simulink model "f16_hifi_euler_vTrim"  (R2020b)
settings: Solver=ode4  StartTime=0.0  StopTime=simTime  FixedStep=stepTime  RelTol=1e-3
undefined symbols (not defined in the file): data, ft, outputs, s
libraries: libAeroLookUpTables x9, aerolibconvert2 x7, lib6DOFUtilityEquations x6, libTFActuatorCalc x5, aerolibtransform2 x1, libEngineAngMomSpecs x1, libAircraftMoISpecs x1, libAircraftWeightandMassSpec x1, libAircraftWingFusalageSpecs x1, libCmdPowConversion x1, libEngineThrustCalc x1, libAtmosphereModel x1
(part 2 of 3)

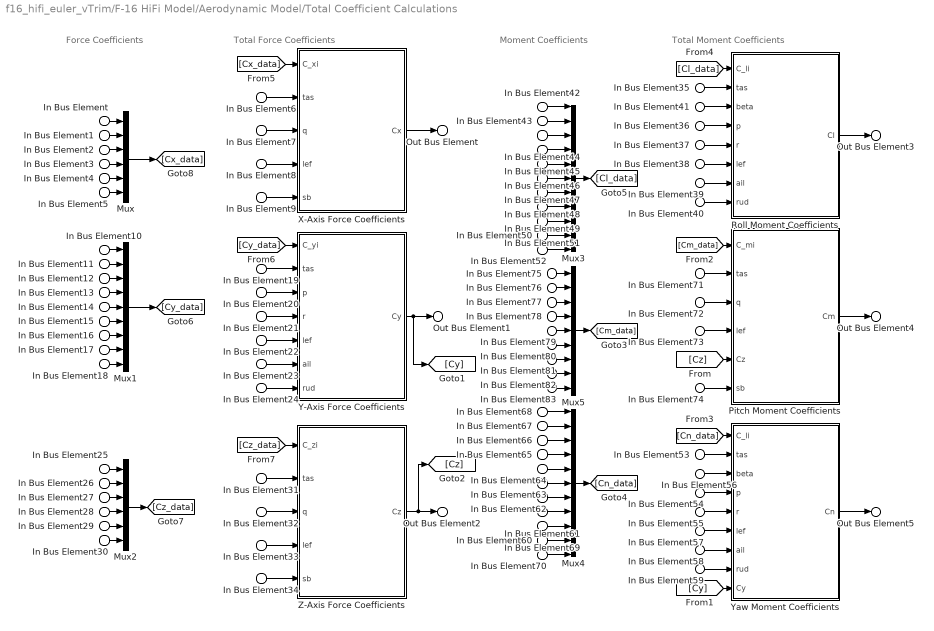
== system f16_hifi_euler_vTrim/F-16 HiFi Model/Aerodynamic Model/Total Coefficient Calculations ==
  note: Total Moment Coefficients
  note: Total Force Coefficients
  note: Force Coefficients
  note: Moment Coefficients
  In Bus Element : Inport  PortName=coeffs  Element=Cx
  In Bus Element1 : Inport  PortName=coeffs  Element=Cxq
  In Bus Element2 : Inport  PortName=coeffs  Element=Cxlef
  In Bus Element3 : Inport  PortName=coeffs  Element=Cxqlef
  In Bus Element4 : Inport  PortName=coeffs  Element=Cxsb
  In Bus Element5 : Inport  PortName=coeffs  Element=Cx0
  In Bus Element10 : Inport  PortName=coeffs  Element=Cy
  In Bus Element11 : Inport  PortName=coeffs  Element=Cyp
  In Bus Element12 : Inport  PortName=coeffs  Element=Cyr
  In Bus Element13 : Inport  PortName=coeffs  Element=Cyail
  In Bus Element14 : Inport  PortName=coeffs  Element=Cyrud
  In Bus Element15 : Inport  PortName=coeffs  Element=Cylef
  In Bus Element16 : Inport  PortName=coeffs  Element=Cyplef
  In Bus Element17 : Inport  PortName=coeffs  Element=Cyrlef
  In Bus Element18 : Inport  PortName=coeffs  Element=Cyaillef
  In Bus Element25 : Inport  PortName=coeffs  Element=Cz
  In Bus Element26 : Inport  PortName=coeffs  Element=Czq
  In Bus Element27 : Inport  PortName=coeffs  Element=Czlef
  In Bus Element28 : Inport  PortName=coeffs  Element=Czqlef
  In Bus Element29 : Inport  PortName=coeffs  Element=Czsb
  In Bus Element30 : Inport  PortName=coeffs  Element=Cz0
  In Bus Element50 : Inport  PortName=coeffs  Element=Claillef
  In Bus Element49 : Inport  PortName=coeffs  Element=Clrlef
  In Bus Element48 : Inport  PortName=coeffs  Element=Clplef
  In Bus Element47 : Inport  PortName=coeffs  Element=Cllef
  In Bus Element46 : Inport  PortName=coeffs  Element=Clrud
  In Bus Element45 : Inport  PortName=coeffs  Element=Clail
  In Bus Element44 : Inport  PortName=coeffs  Element=Clr
  In Bus Element43 : Inport  PortName=coeffs  Element=Clp
  In Bus Element42 : Inport  PortName=coeffs  Element=Cl
  In Bus Element51 : Inport  PortName=coeffs  Element=Clbeta
  In Bus Element52 : Inport  PortName=coeffs  Element=Cl0
  In Bus Element70 : Inport  PortName=coeffs  Element=Cn0
  In Bus Element60 : Inport  PortName=coeffs  Element=Cnaillef
  In Bus Element69 : Inport  PortName=coeffs  Element=Cnbeta
  In Bus Element61 : Inport  PortName=coeffs  Element=Cnrlef
  In Bus Element62 : Inport  PortName=coeffs  Element=Cnplef
  In Bus Element63 : Inport  PortName=coeffs  Element=Cnlef
  In Bus Element64 : Inport  PortName=coeffs  Element=Cnrud
  In Bus Element65 : Inport  PortName=coeffs  Element=Cnail
  In Bus Element66 : Inport  PortName=coeffs  Element=Cnr
  In Bus Element67 : Inport  PortName=coeffs  Element=Cnp
  In Bus Element75 : Inport  PortName=coeffs  Element=Cm
  In Bus Element76 : Inport  PortName=coeffs  Element=Cmq
  In Bus Element77 : Inport  PortName=coeffs  Element=Cmlef
  In Bus Element78 : Inport  PortName=coeffs  Element=Cmqlef
  In Bus Element79 : Inport  PortName=coeffs  Element=Cmeta
  In Bus Element80 : Inport  PortName=coeffs  Element=Cmdiff
  In Bus Element81 : Inport  PortName=coeffs  Element=Cmds
  In Bus Element82 : Inport  PortName=coeffs  Element=Cmsb
  In Bus Element83 : Inport  PortName=coeffs  Element=Cm0
  In Bus Element68 : Inport  PortName=coeffs  Element=Cn
  In Bus Element{6,19,31,35,53,71} (6 alike) : Inport  Port=2  PortName=states  Element=tas
  In Bus Element7 : Inport  Port=2  PortName=states  Element=q
  In Bus Element32 : Inport  Port=2  PortName=states  Element=q
  In Bus Element72 : Inport  Port=2  PortName=states  Element=q
  In Bus Element20 : Inport  Port=2  PortName=states  Element=p
  In Bus Element36 : Inport  Port=2  PortName=states  Element=p
  In Bus Element54 : Inport  Port=2  PortName=states  Element=p
  In Bus Element21 : Inport  Port=2  PortName=states  Element=r
  In Bus Element37 : Inport  Port=2  PortName=states  Element=r
  In Bus Element55 : Inport  Port=2  PortName=states  Element=r
  In Bus Element41 : Inport  Port=2  PortName=states  Element=beta
  In Bus Element56 : Inport  Port=2  PortName=states  Element=beta
  In Bus Element{8,22,33,38,57,73} (6 alike) : Inport  Port=3  PortName=actSignals  Element=lef
  In Bus Element9 : Inport  Port=3  PortName=actSignals  Element=sb
  In Bus Element34 : Inport  Port=3  PortName=actSignals  Element=sb
  In Bus Element74 : Inport  Port=3  PortName=actSignals  Element=sb
  In Bus Element23 : Inport  Port=3  PortName=actSignals  Element=ail
  In Bus Element39 : Inport  Port=3  PortName=actSignals  Element=ail
  In Bus Element58 : Inport  Port=3  PortName=actSignals  Element=ail
  In Bus Element24 : Inport  Port=3  PortName=actSignals  Element=rud
  In Bus Element40 : Inport  Port=3  PortName=actSignals  Element=rud
  In Bus Element59 : Inport  Port=3  PortName=actSignals  Element=rud
  Mux : Mux  Inputs=6
  Mux1 : Mux  Inputs=09
  Mux2 : Mux  Inputs=6
  Mux3 : Mux  Inputs=11
  Mux4 : Mux  Inputs=11
  Mux5 : Mux  Inputs=09
  Pitch Moment Coefficients : Subsystem  mask(Aerodynamic Model -> Total Coefficient Calculations -> Total Pitch Moment Body Aerodynamic Coefficient){cbar=data.acSpec.wing.cbar, xcg=data.acSpec.fusalage.x_cg, xcg_ref=data.acSpec.fusalage.x_cg_ref}
      mask prompts: cbar "Mean Aerodynamic Chord"; xcg "X-axis center of gravity"; xcg_ref "Nominal X-axis center of gravity"
      mask help:
      | Total Pitch Moment Body Aerodynamic Coefficient Calculatior.
      | Aircraft state information and control inputs are used for calculations.
      mask Help:
      | This block is used for obtain total pitch moment coefficient with using state and control inputs.
      | -------------------------------------------------------------------------------------------------------------------------------------------------
      | Inputs of the function:
      | 	Coefficients C_{m}s: Pitch Moment whole aerodynamic coefficients at specific conditions.
      | 	tas: True air speed in [ft/s].
      | 	q: Body axis angular rate (pitch) in [rad/s].
      | 	lef: Leading edge flap deflection in [deg].
      | 	C_{z}: Z-Axis total aeodynamic coefficient.
      | Output of the function:
      | 	C_{m}: Pitch Moment total aerodynamic coefficient.
      | -------------------------------------------------------------------------------------------------------------------------------------------------
      | 	- All equations can be found in Steven's text book. Reference can be found in "literature" subfolder.
      | 	- for question: "cagataysahin44@gmail.com"
      mask Display:
      | port_label('input',1,'C_{m_{i}}','texmode','on');
      | port_label('input',2,'V_{tas}','texmode','on');
      | port_label('input',3,'q','texmode','on');
      | port_label('input',4,'\delta_{lef}','texmode','on');
      | port_label('input',5,'C_{z}','texmode','on');
      | port_label('input',6,'\delta_{sb}','texmode','on');
      | 
      | port_label('output',1,'C_{m}','texmode','on');
  Roll Moment Coefficients : Subsystem  mask(Aerodynamic Model -> Total Coefficient Calculations -> Total Roll Moment Body Aerodynamic Coefficient){b=data.acSpec.wing.b}
      mask prompts: b "Wing Span"
      mask help:
      | Total Roll Moment Aerodynamic Coefficient Calculatior.
      | Aircraft state information and control inputs are used for calculations.
      mask Help:
      | This block is used for obtain total roll moment aerodynamic force coefficient. The equations are taken from Steven's textbook.,
      | -------------------------------------------------------------------------------------------------------------------------------------------------
      | Inputs of the function:
      | 	Coefficients C_{l}s: Roll moment whole aerodynamic coefficients at specific conditions.
      | 	tas: True air speed in [ft/s].
      |  	beta: Sideslip angle in [rad].
      | 	p: Body axis angular rate (roll) in [rad/s].
      | 	r: Body axis angular rate (yaw) in [rad/s].
      | 	lef: Leading edge flap deflection in [deg].
      | 	ail: Aileron deflection in [deg].
      | 	rud: Rudder deflection in [deg].
      | Output of the function:
      | 	C_{l}: Roll moment aerodynamic coefficient.
      | -------------------------------------------------------------------------------------------------------------------------------------------------
      | 	- All equations can be found in Steven's text book. Reference can be found in "literature" subfolder.
      | 	- for question: "cagataysahin44@gmail.com"
      mask Display:
      | port_label('input',1,'C_{l_{i}}','texmode','on');
      | port_label('input',2,'V_{tas}','texmode','on');
      | port_label('input',3,'\beta','texmode','on');
      | port_label('input',4,'p','texmode','on');
      | port_label('input',5,'r','texmode','on');
      | port_label('input',6,'\delta_{lef}','texmode','on');
      | port_label('input',7,'\delta_{ail}','texmode','on');
      | port_label('input',8,'\delta_{rud}','texmode','on');
      | 
      | port_label('output',1,'C_{l}','texmode','on');
  X-Axis Force Coefficients : Subsystem  mask(Aerodynamic Model -> Total Coefficient Calculations -> Total X-Axis Body Aerodynamic Coefficient){cbar=data.acSpec.wing.cbar}
      mask prompts: cbar "Mean Aerodynamic Chord"
      mask help:
      | Total X-Axis Body Aerodynamic Coefficient Calculatior.
      | Aircraft state information and control inputs are used for calculations.
      mask Help:
      | This block is used for obtain total x-axis aerodynamic force coefficient with using state and control inputs.
      | -------------------------------------------------------------------------------------------------------------------------------------------------
      | Inputs of the function:
      | 	Coefficients C_{x}s: X-Axis whole aerodynamic coefficients at specific conditions.
      | 	tas: True air speed in [ft/s].
      | 	q: Body axis angular rate (pitch) in [rad/s].
      | 	lef: Leading edge flap deflection in [deg].
      | Output of the function:
      | 	C_{x}: X-Axis total aerodynamic coefficient.
      | -------------------------------------------------------------------------------------------------------------------------------------------------
      | 	- All equations can be found in Steven's text book. Reference can be found in "literature" subfolder.
      | 	- for question: "cagataysahin44@gmail.com"
      mask Display:
      | port_label('input',1,'C_{x_{i}}','texmode','on');
      | port_label('input',2,'V_{tas}','texmode','on');
      | port_label('input',3,'q','texmode','on');
      | port_label('input',4,'\delta_{lef}','texmode','on');
      | port_label('input',5,'\delta_{sb}','texmode','on');
      | 
      | port_label('output',1,'C_{x}','texmode','on');
  Y-Axis Force Coefficients : Subsystem  mask(Aerodynamic Model -> Total Coefficient Calculations -> Total Y-Axis Body Aerodynamic Coefficient){b=data.acSpec.wing.b}
      mask prompts: b "Wing Span"
      mask help:
      | Total Y-Axis Body Aerodynamic Coefficient Calculatior.
      | Aircraft state information and control inputs are used for calculations.
      mask Help:
      | This block is used for obtain total x-axis aerodynamic force coefficient with using state and control inputs.
      | -------------------------------------------------------------------------------------------------------------------------------------------------
      | Inputs of the function:
      | 	Coefficients C_{y}s: Y-Axis whole aerodynamic coefficients at specific conditions.
      | 	tas: True air speed in [ft/s].
      | 	p: Body axis angular rate (y-axis) in [rad/s].
      | 	r: Body axis angular rate (y-axis) in [rad/s].
      | 	lef: Leading edge flap deflection in [deg].
      | 	ail: Aileron deflection in [deg].
      | 	rud: Rudder deflection in [deg].
      | Output of the function:
      | 	C_{y}: Y-axis total aerodynamic coefficient.
      | -------------------------------------------------------------------------------------------------------------------------------------------------
      | 	- All equations can be found in Steven's text book. Reference can be found in "literature" subfolder.
      | 	- for question: "cagataysahin44@gmail.com"
      mask Display:
      | port_label('input',1,'C_{y_{i}}','texmode','on');
      | port_label('input',2,'V_{tas}','texmode','on');
      | port_label('input',3,'p','texmode','on');
      | port_label('input',4,'r','texmode','on');
      | port_label('input',5,'\delta_{lef}','texmode','on');
      | port_label('input',6,'\delta_{ail}','texmode','on');
      | port_label('input',7,'\delta_{rud}','texmode','on');
      | 
      | port_label('output',1,'C_{y}','texmode','on');
  Yaw Moment Coefficients : Subsystem  mask(Aerodynamic Model -> Total Coefficient Calculations -> Total Yaw Moment Body Aerodynamic Coefficient){b=data.acSpec.wing.b, xcg=data.acSpec.fusalage.x_cg, xcg_ref=data.acSpec.fusalage.x_cg_ref, cbar=data.acSpec.wing.cbar}
      mask prompts: b "Wing Span"; xcg "Center of Gravity"; xcg_ref "Nominal Center of Gravity"; cbar "Mean Aerodynamic Chord"
      mask help:
      | Total Yaw Moment Aerodynamic Coefficient Calculatior.
      | Aircraft state information and control inputs are used for calculations.
      mask Help:
      | This block is used for obtain total yaw moment aerodynamic force coefficient. The equations are taken from Steven's textbook.,
      | -------------------------------------------------------------------------------------------------------------------------------------------------
      | Inputs of the function:
      | 	Coefficients C_{n}s: Yaw moment whole aerodynamic coefficients at specific conditions.
      | 	tas: True air speed in [ft/s].
      |  	beta: Sideslip angle in [rad].
      | 	p: Body axis angular rate (roll) in [rad/s].
      | 	r: Body axis angular rate (yaw) in [rad/s].
      | 	lef: Leading edge flap deflection in [deg].
      | 	ail: Aileron deflection in [deg].
      | 	rud: Rudder deflection in [deg].
      | 	C_{y}: Total Y-Axis aerodynamic coefficient.
      | Output of the function:
      | 	C_{n}: Yaw moment aerodynamic coefficient.
      | -------------------------------------------------------------------------------------------------------------------------------------------------
      | 	- All equations can be found in Steven's text book. Reference can be found in "literature" subfolder.
      | 	- for question: "cagataysahin44@gmail.com"
      mask Display:
      | port_label('input',1,'C_{n_{i}}','texmode','on');
      | port_label('input',2,'V_{tas}','texmode','on');
      | port_label('input',3,'\beta','texmode','on');
      | port_label('input',4,'p','texmode','on');
      | port_label('input',5,'r','texmode','on');
      | port_label('input',6,'\delta_{lef}','texmode','on');
      | port_label('input',7,'\delta_{ail}','texmode','on');
      | port_label('input',8,'\delta_{rud}','texmode','on');
      | port_label('input',9,'C_{y}','texmode','on');
      | 
      | port_label('output',1,'C_{n}','texmode','on');
  Z-Axis Force Coefficients : Subsystem  mask(Aerodynamic Model -> Total Coefficient Calculations -> Total Z-Axis Body Aerodynamic Coefficient){cbar=data.acSpec.wing.cbar}
      mask prompts: cbar "Mean Aerodynamic Chord"
      mask help:
      | Total Z-Axis Body Aerodynamic Coefficient Calculatior.
      | Aircraft state information and control inputs are used for calculations.
      mask Help:
      | This block is used for obtain total z-axis aerodynamic force coefficient with using state and control inputs.
      | -------------------------------------------------------------------------------------------------------------------------------------------------
      | Inputs of the function:
      | 	Coefficients C_{z}s: Z-Axis whole aerodynamic coefficients at specific conditions.
      | 	tas: True air speed in [ft/s].
      | 	q: Body axis angular rate (pitch) in [rad/s].
      | 	lef: Leading edge flap deflection in [deg].
      | Output of the function:
      | 	C_{z}: X-Axis total aerodynamic coefficient.
      | -------------------------------------------------------------------------------------------------------------------------------------------------
      | 	- All equations can be found in Steven's text book. Reference can be found in "literature" subfolder.
      | 	- for question: "cagataysahin44@gmail.com"
      mask Display:
      | port_label('input',1,'C_{z_{i}}','texmode','on');
      | port_label('input',2,'V_{tas}','texmode','on');
      | port_label('input',3,'q','texmode','on');
      | port_label('input',4,'\delta_{lef}','texmode','on');
      | port_label('input',5,'\delta_{sb}','texmode','on');
      | 
      | port_label('output',1,'C_{z}','texmode','on');
  Out Bus Element : Outport  PortName=totalCoeffs  Element=Cx
  Out Bus Element1 : Outport  PortName=totalCoeffs  Element=Cy
  Out Bus Element2 : Outport  PortName=totalCoeffs  Element=Cz
  Out Bus Element3 : Outport  PortName=totalCoeffs  Element=Cl
  Out Bus Element4 : Outport  PortName=totalCoeffs  Element=Cm
  Out Bus Element5 : Outport  PortName=totalCoeffs  Element=Cn
  wires:
  In Bus Element17/1 -> Mux1/8
  In Bus Element78/1 -> Mux5/4
  X-Axis Force Coefficients/1(Cx) -> Out Bus Element/1
  In Bus Element74/1 -> Pitch Moment Coefficients/6(sb)
  In Bus Element23/1 -> Y-Axis Force Coefficients/6(ail)
  In Bus Element7/1 -> X-Axis Force Coefficients/3(q)
  In Bus Element83/1 -> Mux5/9
  In Bus Element68/1 -> Mux4/1
  In Bus Element80/1 -> Mux5/6
  In Bus Element35/1 -> Roll Moment Coefficients/2(tas)
  In Bus Element54/1 -> Yaw Moment Coefficients/4(p)
  In Bus Element44/1 -> Mux3/3
  In Bus Element22/1 -> Y-Axis Force Coefficients/5(lef)
  Y-Axis Force Coefficients/1(Cy) -> [Cy], Out Bus Element1/1
  In Bus Element29/1 -> Mux2/5
  In Bus Element30/1 -> Mux2/6
  In Bus Element1/1 -> Mux/2
  In Bus Element57/1 -> Yaw Moment Coefficients/6(lef)
  In Bus Element73/1 -> Pitch Moment Coefficients/4(lef)
  In Bus Element43/1 -> Mux3/2
  In Bus Element20/1 -> Y-Axis Force Coefficients/3(p)
  In Bus Element59/1 -> Yaw Moment Coefficients/8(rud)
  In Bus Element77/1 -> Mux5/3
  In Bus Element82/1 -> Mux5/8
  In Bus Element24/1 -> Y-Axis Force Coefficients/7(rud)
  In Bus Element2/1 -> Mux/3
  In Bus Element63/1 -> Mux4/6
  In Bus Element69/1 -> Mux4/9
  In Bus Element45/1 -> Mux3/4
  In Bus Element3/1 -> Mux/4
  Roll Moment Coefficients/1(Cl) -> Out Bus Element3/1
  In Bus Element38/1 -> Roll Moment Coefficients/6(lef)
  In Bus Element5/1 -> Mux/6
  In Bus Element61/1 -> Mux4/8
  In Bus Element15/1 -> Mux1/6
  In Bus Element4/1 -> Mux/5
  In Bus Element37/1 -> Roll Moment Coefficients/5(r)
  In Bus Element53/1 -> Yaw Moment Coefficients/2(tas)
  In Bus Element27/1 -> Mux2/3
  Mux5/1 -> [Cm_data]
  In Bus Element18/1 -> Mux1/9
  In Bus Element60/1 -> Mux4/10
  In Bus Element14/1 -> Mux1/5
  In Bus Element55/1 -> Yaw Moment Coefficients/5(r)
  In Bus Element31/1 -> Z-Axis Force Coefficients/2(tas)
  In Bus Element81/1 -> Mux5/7
  In Bus Element49/1 -> Mux3/8
  In Bus Element39/1 -> Roll Moment Coefficients/7(ail)
  In Bus Element34/1 -> Z-Axis Force Coefficients/5(sb)
  In Bus Element13/1 -> Mux1/4
  In Bus Element32/1 -> Z-Axis Force Coefficients/3(q)
  In Bus Element70/1 -> Mux4/11
  In Bus Element21/1 -> Y-Axis Force Coefficients/4(r)
  In Bus Element50/1 -> Mux3/10
  In Bus Element10/1 -> Mux1/1
  Z-Axis Force Coefficients/1(Cz) -> [Cz], Out Bus Element2/1
  In Bus Element42/1 -> Mux3/1
  In Bus Element8/1 -> X-Axis Force Coefficients/4(lef)
  In Bus Element67/1 -> Mux4/2
  Pitch Moment Coefficients/1(Cm) -> Out Bus Element4/1
  In Bus Element46/1 -> Mux3/5
  In Bus Element64/1 -> Mux4/5
  In Bus Element79/1 -> Mux5/5
  In Bus Element19/1 -> Y-Axis Force Coefficients/2(tas)
  In Bus Element52/1 -> Mux3/11
  In Bus Element62/1 -> Mux4/7
  In Bus Element47/1 -> Mux3/6
  In Bus Element48/1 -> Mux3/7
  In Bus Element76/1 -> Mux5/2
  In Bus Element16/1 -> Mux1/7
  In Bus Element71/1 -> Pitch Moment Coefficients/2(tas)
  In Bus Element33/1 -> Z-Axis Force Coefficients/4(lef)
  In Bus Element6/1 -> X-Axis Force Coefficients/2(tas)
  In Bus Element28/1 -> Mux2/4
  In Bus Element26/1 -> Mux2/2
  In Bus Element40/1 -> Roll Moment Coefficients/8(rud)
  In Bus Element51/1 -> Mux3/9
  Yaw Moment Coefficients/1(Cn) -> Out Bus Element5/1
  In Bus Element9/1 -> X-Axis Force Coefficients/5(sb)
  In Bus Element11/1 -> Mux1/2
  In Bus Element25/1 -> Mux2/1
  In Bus Element58/1 -> Yaw Moment Coefficients/7(ail)
  In Bus Element36/1 -> Roll Moment Coefficients/4(p)
  In Bus Element72/1 -> Pitch Moment Coefficients/3(q)
  In Bus Element/1 -> Mux/1
  In Bus Element56/1 -> Yaw Moment Coefficients/3(beta)
  In Bus Element66/1 -> Mux4/3
  In Bus Element41/1 -> Roll Moment Coefficients/3(beta)
  In Bus Element12/1 -> Mux1/3
  In Bus Element75/1 -> Mux5/1
  In Bus Element65/1 -> Mux4/4
  [Cz] -> Pitch Moment Coefficients/5(Cz)
  [Cy] -> Yaw Moment Coefficients/9(Cy)
  [Cm_data] -> Pitch Moment Coefficients/1(C_mi)
  Mux4/1 -> [Cn_data]
  [Cn_data] -> Yaw Moment Coefficients/1(C_li)
  Mux3/1 -> [Cl_data]
  [Cl_data] -> Roll Moment Coefficients/1(C_li)
  Mux/1 -> [Cx_data]
  Mux1/1 -> [Cy_data]
  Mux2/1 -> [Cz_data]
  [Cx_data] -> X-Axis Force Coefficients/1(C_xi)
  [Cy_data] -> Y-Axis Force Coefficients/1(C_yi)
  [Cz_data] -> Z-Axis Force Coefficients/1(C_zi)

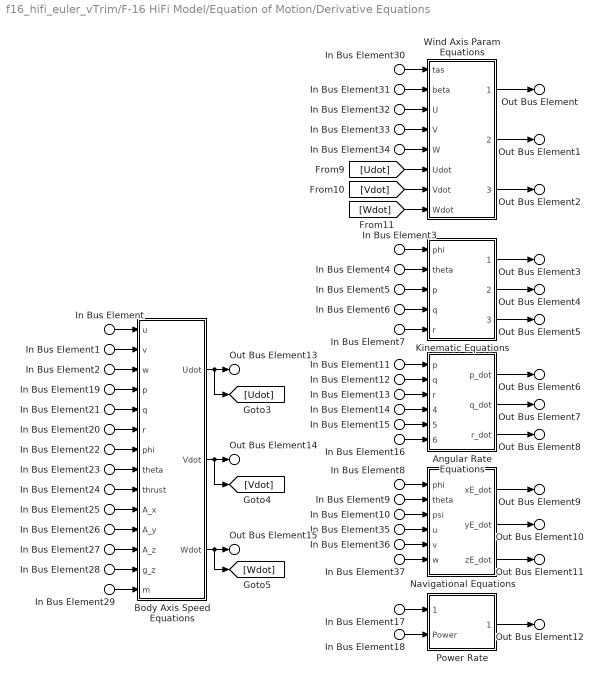
== system f16_hifi_euler_vTrim/F-16 HiFi Model/Equation of Motion/Derivative Equations ==
  In Bus Element30 : Inport  PortName=states  Element=tas
  In Bus Element31 : Inport  PortName=states  Element=beta
  In Bus Element3 : Inport  PortName=states  Element=phi
  In Bus Element8 : Inport  PortName=states  Element=phi
  In Bus Element22 : Inport  PortName=states  Element=phi
  In Bus Element4 : Inport  PortName=states  Element=theta
  In Bus Element9 : Inport  PortName=states  Element=theta
  In Bus Element23 : Inport  PortName=states  Element=theta
  In Bus Element5 : Inport  PortName=states  Element=p
  In Bus Element11 : Inport  PortName=states  Element=p
  In Bus Element19 : Inport  PortName=states  Element=p
  In Bus Element7 : Inport  PortName=states  Element=r
  In Bus Element13 : Inport  PortName=states  Element=r
  In Bus Element20 : Inport  PortName=states  Element=r
  In Bus Element10 : Inport  PortName=states  Element=psi
  In Bus Element6 : Inport  PortName=states  Element=q
  In Bus Element12 : Inport  PortName=states  Element=q
  In Bus Element21 : Inport  PortName=states  Element=q
  In Bus Element18 : Inport  PortName=states  Element=power
  In Bus Element14 : Inport  Port=2  PortName=aeroFM  Element=L
  In Bus Element15 : Inport  Port=2  PortName=aeroFM  Element=M
  In Bus Element16 : Inport  Port=2  PortName=aeroFM  Element=N
  In Bus Element25 : Inport  Port=2  PortName=aeroFM  Element=X
  In Bus Element26 : Inport  Port=2  PortName=aeroFM  Element=Y
  In Bus Element27 : Inport  Port=2  PortName=aeroFM  Element=Z
  In Bus Element17 : Inport  Port=3  PortName=engine  Element=cmdPow
  In Bus Element24 : Inport  Port=3  PortName=engine  Element=thrust
  In Bus Element28 : Inport  Port=4  PortName=graParam  Element=g_z
  In Bus Element29 : Inport  Port=5  PortName=acSpecs  Element=m
  In Bus Element : Inport  Port=6  PortName=sensorData  Element=u
  In Bus Element32 : Inport  Port=6  PortName=sensorData  Element=u
  In Bus Element35 : Inport  Port=6  PortName=sensorData  Element=u
  In Bus Element1 : Inport  Port=6  PortName=sensorData  Element=v
  In Bus Element33 : Inport  Port=6  PortName=sensorData  Element=v
  In Bus Element36 : Inport  Port=6  PortName=sensorData  Element=v
  In Bus Element2 : Inport  Port=6  PortName=sensorData  Element=w
  In Bus Element34 : Inport  Port=6  PortName=sensorData  Element=w
  In Bus Element37 : Inport  Port=6  PortName=sensorData  Element=w
  Angular Rate Equations : Subsystem  mask(Equation of Motion - CAME (Angular Rate) Equations.){I_xx=data.acSpec.inertia.I_xx, I_yy=data.acSpec.inertia.I_yy, I_zz=data.acSpec.inertia.I_zz, I_xz=data.acSpec.inertia.I_xz, h_x=data.engine.specs.angMom.h_x}
      mask prompts: I_xx "Inertia on X-axis"; I_yy "Inertia on Y-axis"; I_zz "Inertia on Z-axis"; I_xz "Inertia on XZ-axis"; h_x "Angular Momentum on X-axis"
      mask help: Aircraft Conversation of Angular Momentum Equation which calculates angular rates.
      mask Help:
      | Aircraft Conversation of Angular Momentum Equation which calculates angular rates which using moment and state information as an input.
      | -------------------------------------------------------------------------------------------------------------------------------------------------
      | Inputs of this block:
      | 	Body Axis Speed: U, V, W information [ft/s].
      | 	Body Axis Moments: M_l, M_M, M_N information
      | Outputs of this block:
      | 	Ang. Rates Der.: Derivative of Angular Rates [rad/sec^2].
      | -------------------------------------------------------------------------------------------------------------------------------------------------
      | 	- Equations that in this block can be found in Steven's textbook. This textbook is in "literature" subfolder.
      | 	- for question: "cagataysahin44@gmail.com".
      mask Display:
      | port_label('input',1,'p','texmode','on');
      | port_label('input',2,'q','texmode','on');
      | port_label('input',3,'r','texmode','on');
      | port_label('input',4,'M_{L}','texmode','on');
      | port_label('input',5,'M_{M}','texmode','on');
      | port_label('input',6,'M_{N}','texmode','on');
      | 
      | port_label('output',1,'p_{der}','texmode','on');
      | port_label('output',2,'q_{der}','texmode','on');
      | port_label('output',3,'r_{der}','texmode','on');
  Body Axis Speed Equations : Subsystem  mask(EOM Model - Body Axis Speed Equations){}
      mask help: Aircraft body axis speeds calculation equations.
      mask Help:
      | This block can calculate aircraft's body axis speeds with using state, thrust, force and gravity information.
      | -------------------------------------------------------------------------------------------------------------------------------------------------
      | Inputs of this block:
      | 	Euler Angles: Roll, Pitch information [rad].
      | 	Body Axis Speed: U, V, W information [ft/s].
      | 	T: Thrust information [lbf].
      | 	A_{i}: Aerodynamic force information [lbf].
      | 	g: gravity information [ft/sec^2].
      | 	m: Aircraft Mass [slug].
      | Outputs of this block:
      | 	Body Axis Speed Ders. Derivative of body axis speeds [ft/sec^2].
      | -------------------------------------------------------------------------------------------------------------------------------------------------
      | 	- Equations that in this block can be found in Steven's textbook. This textbook is in "literature" subfolder.
      | 	- for question: "cagataysahin44@gmail.com".
      mask Display:
      | port_label('input',1,'U','texmode','on');
      | port_label('input',2,'V','texmode','on');
      | port_label('input',3,'W','texmode','on');
      | port_label('input',4,'p','texmode','on');
      | port_label('input',5,'q','texmode','on');
      | port_label('input',6,'r','texmode','on');
      | port_label('input',7,'\phi','texmode','on');
      | port_label('input',8,'\theta','texmode','on');
      | port_label('input',9,'T','texmode','on');
      | port_label('input',10,'A_{x}','texmode','on');
      | port_label('input',11,'A_{y}','texmode','on');
      | port_label('input',12,'A_{z}','texmode','on');
      | port_label('input',13,'g_{z}','texmode','on');
      | port_label('input',14,'m','texmode','on');
      | 
      | port_label('output',1,'U_{der}','texmode','on');
      | port_label('output',2,'V_{der}','texmode','on');
      | port_label('output',3,'W_{der}','texmode','on');
  Kinematic Equations : Subsystem  mask(Equation of Motion - Kinematic Equation for Euler Angles.){}
      mask help: Aircraft kinematic equtions which is in Euler Angles form.
      mask Help:
      | This block can calculate aircaft's kinematic parameters in Euler Angles form.
      | -------------------------------------------------------------------------------------------------------------------------------------------------
      | Inputs of this block:
      | 	Euler Angles: Roll, Pitch, information [rad].
      | 	Body Axis Angular Rates: p, q, r information [rad/s].
      | Outputs of this block:
      | 	Euler Angles Ders: Derivative of Euler Angles.
      | -------------------------------------------------------------------------------------------------------------------------------------------------
      | 	- Equations that in this block can be found in Steven's textbook. This textbook is in "literature" subfolder.
      | 	- for question: "cagataysahin44@gmail.com".
      mask Display:
      | port_label('input',1,'\phi','texmode','on');
      | port_label('input',2,'\theta','texmode','on');
      | port_label('input',3,'p','texmode','on');
      | port_label('input',4,'q','texmode','on');
      | port_label('input',5,'r','texmode','on');
      | 
      | port_label('output',1,'\phi_{der}','texmode','on');
      | port_label('output',2,'\theta_{der}','texmode','on');
      | port_label('output',3,'\psi_{der}','texmode','on');
  Navigational Equations : Subsystem  mask(EOM Model - Navigational Equations){}
      mask help: Aircraft navigational equations which is known as flight path.
      mask Help:
      | This block can calculate aircaft's flight path information with using state inputs.
      | -------------------------------------------------------------------------------------------------------------------------------------------------
      | Inputs of this block:
      | 	Euler Angles: Roll, Pitch, Yaw information [rad].
      | 	Body Axis Speed: U, V, W information [ft/s].
      | Outputs of this block:
      | 	p_{e}: Derivative of position of aircraft in NED Coordinate System [ft].
      | -------------------------------------------------------------------------------------------------------------------------------------------------
      | 	- Equations that in this block can be found in Steven's textbook. This textbook is in "literature" subfolder.
      | 	- for question: "cagataysahin44@gmail.com".
      mask Display:
      | port_label('input',1,'\phi','texmode','on');
      | port_label('input',2,'\theta','texmode','on');
      | port_label('input',3,'\psi','texmode','on');
      | port_label('input',4,'u','texmode','on');
      | port_label('input',5,'v','texmode','on');
      | port_label('input',6,'w','texmode','on');
      | 
      | port_label('output',1,'x_{e_{der}}','texmode','on');
      | port_label('output',2,'y_{e_{der}}','texmode','on');
      | port_label('output',3,'z_{e_{der}}','texmode','on');
  Power Rate : Subsystem  mask(EOM Model - Power Rate Calculation){}
      mask help:
      | Power Rate Calculation
      | Calculate actual power output with using initial trim values and commanded power values.
      | All works can be found in Steven's examples. References can be found in "literature".
      mask Help:
      | Power Rate Calculation
      | ----------------------------------
      | 	Inputs => Commanded Power
      | 	Outputs => Actual Power
      | ----------------------------------
      | for question "cagataysahin44@gmail.com".
      mask Display:
      | port_label('input',1,'Pow_{cmd}','texmode','on');
      | port_label('input',2,'Pow_{act}','texmode','on');
      | 
      | port_label('output',1,'der_{Pow_{act}}','texmode','on');
  Wind Axis Param Equations : Subsystem  mask(EOM Model - Wind Axis Paramater Equations.){}
      mask help: Aircraft wind parameter information calculation which is angle of attack, angle of sideslip and true airspeed.
      mask Help:
      | This block can calculate aircaft's wind parameters which using state inputs.
      | -------------------------------------------------------------------------------------------------------------------------------------------------
      | Inputs of this block:
      | 	Wind Params: True airspeed, AoA and AoS [ft/s, rad].
      | 	Body Speeds: U, V, W information [ft/s].
      | 	Body Speed Ders: U, V, W derivative information [ft/sec^2].
      | Outputs of this block:
      | 	Wind Param Ders: Derivative information of wind parameters. [ft/sec^2, rad/sec].
      | -------------------------------------------------------------------------------------------------------------------------------------------------
      | 	- Equations that in this block can be found in Steven's textbook. This textbook is in "literature" subfolder.
      | 	- for question: "cagataysahin44@gmail.com".
      mask Display:
      | port_label('input',1,'V_{tas}','texmode','on');
      | port_label('input',2,'\beta','texmode','on');
      | port_label('input',3,'U','texmode','on');
      | port_label('input',4,'V','texmode','on');
      | port_label('input',5,'W','texmode','on');
      | port_label('input',6,'U_{der}','texmode','on');
      | port_label('input',7,'V_{der}','texmode','on');
      | port_label('input',8,'W_{der}','texmode','on');
      | 
      | port_label('output',1,'V_{tas_{der}}','texmode','on');
      | port_label('output',2,'\alpha_{der}','texmode','on');
      | port_label('output',3,'\beta_{der}','texmode','on');
  Out Bus Element : Outport  PortName=ders  Element=tas
  Out Bus Element1 : Outport  PortName=ders  Element=alpha
  Out Bus Element2 : Outport  PortName=ders  Element=beta
  Out Bus Element3 : Outport  PortName=ders  Element=phi
  Out Bus Element4 : Outport  PortName=ders  Element=theta
  Out Bus Element5 : Outport  PortName=ders  Element=psi
  Out Bus Element6 : Outport  PortName=ders  Element=p
  Out Bus Element7 : Outport  PortName=ders  Element=q
  Out Bus Element8 : Outport  PortName=ders  Element=r
  Out Bus Element9 : Outport  PortName=ders  Element=x_e
  Out Bus Element10 : Outport  PortName=ders  Element=y_e
  Out Bus Element11 : Outport  PortName=ders  Element=z_e
  Out Bus Element12 : Outport  PortName=ders  Element=power
  Out Bus Element13 : Outport  PortName=ders  Element=u
  Out Bus Element14 : Outport  PortName=ders  Element=v
  Out Bus Element15 : Outport  PortName=ders  Element=w
  wires:
  Wind Axis Param Equations/2(alpha_dot) -> Out Bus Element1/1
  Angular Rate Equations/2(q_dot) -> Out Bus Element7/1
  Angular Rate Equations/1(p_dot) -> Out Bus Element6/1
  In Bus Element3/1 -> Kinematic Equations/1("phi ")
  In Bus Element2/1 -> Body Axis Speed Equations/3(w)
  Navigational Equations/2(yE_dot) -> Out Bus Element10/1
  Navigational Equations/3(zE_dot) -> Out Bus Element11/1
  In Bus Element20/1 -> Body Axis Speed Equations/6(r)
  In Bus Element12/1 -> Angular Rate Equations/2(q)
  Kinematic Equations/1(phi_dot) -> Out Bus Element3/1
  In Bus Element15/1 -> Angular Rate Equations/5(aeroM_M)
  In Bus Element8/1 -> Navigational Equations/1("phi ")
  In Bus Element/1 -> Body Axis Speed Equations/1(u)
  Angular Rate Equations/3(r_dot) -> Out Bus Element8/1
  Kinematic Equations/3(psi_dot) -> Out Bus Element5/1
  In Bus Element5/1 -> Kinematic Equations/3(p)
  Wind Axis Param Equations/1(tas_dot) -> Out Bus Element/1
  [Vdot] -> Wind Axis Param Equations/7(Vdot)
  Navigational Equations/1(xE_dot) -> Out Bus Element9/1
  [Wdot] -> Wind Axis Param Equations/8(Wdot)
  Wind Axis Param Equations/3(beta_dot) -> Out Bus Element2/1
  In Bus Element23/1 -> Body Axis Speed Equations/8(theta)
  In Bus Element29/1 -> Body Axis Speed Equations/14(m)
  In Bus Element21/1 -> Body Axis Speed Equations/5(q)
  Body Axis Speed Equations/3(Wdot) -> Out Bus Element15/1, [Wdot]
  In Bus Element30/1 -> Wind Axis Param Equations/1(tas)
  In Bus Element1/1 -> Body Axis Speed Equations/2(v)
  In Bus Element32/1 -> Wind Axis Param Equations/3(U)
  In Bus Element35/1 -> Navigational Equations/4(u)
  In Bus Element36/1 -> Navigational Equations/5(v)
  In Bus Element31/1 -> Wind Axis Param Equations/2(beta)
  In Bus Element28/1 -> Body Axis Speed Equations/13(g_z)
  In Bus Element7/1 -> Kinematic Equations/5(r)
  Power Rate/1(powerDot) -> Out Bus Element12/1
  In Bus Element10/1 -> Navigational Equations/3(psi)
  In Bus Element17/1 -> Power Rate/1(commanded Power)
  In Bus Element22/1 -> Body Axis Speed Equations/7(phi)
  In Bus Element18/1 -> Power Rate/2(Power)
  In Bus Element25/1 -> Body Axis Speed Equations/10(A_x)
  In Bus Element16/1 -> Angular Rate Equations/6(aeroM_N)
  In Bus Element14/1 -> Angular Rate Equations/4(aeroM_L)
  In Bus Element9/1 -> Navigational Equations/2(theta)
  In Bus Element34/1 -> Wind Axis Param Equations/5(W)
  [Udot] -> Wind Axis Param Equations/6(Udot)
  In Bus Element37/1 -> Navigational Equations/6(w)
  In Bus Element27/1 -> Body Axis Speed Equations/12(A_z)
  In Bus Element33/1 -> Wind Axis Param Equations/4(V)
  In Bus Element11/1 -> Angular Rate Equations/1(p)
  In Bus Element19/1 -> Body Axis Speed Equations/4(p)
  Body Axis Speed Equations/1(Udot) -> Out Bus Element13/1, [Udot]
  In Bus Element24/1 -> Body Axis Speed Equations/9(thrust)
  In Bus Element13/1 -> Angular Rate Equations/3(r)
  In Bus Element26/1 -> Body Axis Speed Equations/11(A_y)
  Kinematic Equations/2(theta_dot) -> Out Bus Element4/1
  In Bus Element4/1 -> Kinematic Equations/2(theta)
  In Bus Element6/1 -> Kinematic Equations/4(q)
  Body Axis Speed Equations/2(Vdot) -> Out Bus Element14/1, [Vdot]

== system f16_hifi_euler_vTrim/F-16 HiFi Model/Equation of Motion/Utility Functions ==
  In Bus Element : Inport  PortName=states  Element=tas
  In Bus Element18 : Inport  PortName=states  Element=tas
  In Bus Element1 : Inport  PortName=states  Element=alpha
  In Bus Element19 : Inport  PortName=states  Element=alpha
  In Bus Element2 : Inport  PortName=states  Element=beta
  In Bus Element3 : Inport  PortName=states  Element=phi
  In Bus Element11 : Inport  PortName=states  Element=phi
  In Bus Element4 : Inport  PortName=states  Element=theta
  In Bus Element12 : Inport  PortName=states  Element=theta
  In Bus Element5 : Inport  PortName=states  Element=p
  In Bus Element20 : Inport  PortName=states  Element=p
  In Bus Element6 : Inport  PortName=states  Element=q
  In Bus Element7 : Inport  PortName=states  Element=r
  In Bus Element21 : Inport  PortName=states  Element=r
  In Bus Element13 : Inport  PortName=states  Element=psi
  In Bus Element14 : Inport  PortName=states  Element=x_e
  In Bus Element15 : Inport  PortName=states  Element=y_e
  In Bus Element16 : Inport  PortName=states  Element=z_e
  In Bus Element17 : Inport  PortName=states  Element=z_e
  In Bus Element8 : Inport  Port=2  PortName=graParam  Element=g_z
  In Bus Element9 : Inport  Port=3  PortName=ders  Element=v
  In Bus Element10 : Inport  Port=3  PortName=ders  Element=w
  Acceleration Sensor : lib6DOFUtilityEquations/Acceleration Sensor
      settings: SourceProductName=F16 Aircraft Sub System Models
  Body Axes Rates to Stability Axes Rates : lib6DOFUtilityEquations/Body Axes Rates to Stability Axes Rates
      settings: SourceProductName=F16 Aircraft Sub System Models
  Body Axis Speeds : lib6DOFUtilityEquations/Body Axis Speeds
      settings: SourceProductName=F16 Aircraft Sub System Models
  Euler to Quaternions : lib6DOFUtilityEquations/Euler to Quaternions
      settings: SourceProductName=F16 Aircraft Sub System Models
  NED to LLA Transformation : lib6DOFUtilityEquations/NED to LLA Transformation
      settings: SourceProductName=F16 Aircraft Sub System Models
  True Airspeed to Indicated Airspeed : lib6DOFUtilityEquations/True Airspeed to Indicated Airspeed
      settings: SourceProductName=F16 Aircraft Sub System Models
  Out Bus Element : Outport  PortName=sensorData  Element=u
  Out Bus Element1 : Outport  PortName=sensorData  Element=v
  Out Bus Element2 : Outport  PortName=sensorData  Element=w
  Out Bus Element3 : Outport  PortName=sensorData  Element=aN
  Out Bus Element4 : Outport  PortName=sensorData  Element=aY
  Out Bus Element5 : Outport  PortName=sensorData  Element=q0
  Out Bus Element6 : Outport  PortName=sensorData  Element=q1
  Out Bus Element7 : Outport  PortName=sensorData  Element=q2
  Out Bus Element8 : Outport  PortName=sensorData  Element=q3
  Out Bus Element9 : Outport  PortName=sensorData  Element=lat
  Out Bus Element10 : Outport  PortName=sensorData  Element=long
  Out Bus Element11 : Outport  PortName=sensorData  Element=ias
  Out Bus Element12 : Outport  PortName=sensorData  Element=p_s
  Out Bus Element13 : Outport  PortName=sensorData  Element=r_s
  wires:
  In Bus Element/1 -> Body Axis Speeds/1
  Body Axis Speeds/2 -> Out Bus Element1/1, [v]
  In Bus Element1/1 -> Body Axis Speeds/2
  In Bus Element2/1 -> Body Axis Speeds/3
  Body Axis Speeds/3 -> [w], Out Bus Element2/1
  Body Axis Speeds/1 -> [u], Out Bus Element/1
  [u] -> Acceleration Sensor/1
  [w] -> Acceleration Sensor/3
  [v] -> Acceleration Sensor/2
  In Bus Element3/1 -> Acceleration Sensor/4
  In Bus Element4/1 -> Acceleration Sensor/5
  In Bus Element7/1 -> Acceleration Sensor/8
  In Bus Element6/1 -> Acceleration Sensor/7
  In Bus Element5/1 -> Acceleration Sensor/6
  In Bus Element8/1 -> Acceleration Sensor/9
  In Bus Element10/1 -> Acceleration Sensor/11
  In Bus Element9/1 -> Acceleration Sensor/10
  Acceleration Sensor/1 -> Out Bus Element3/1
  Acceleration Sensor/2 -> Out Bus Element4/1
  In Bus Element11/1 -> Euler to Quaternions/1
  In Bus Element12/1 -> Euler to Quaternions/2
  In Bus Element13/1 -> Euler to Quaternions/3
  Euler to Quaternions/4 -> Out Bus Element8/1
  Euler to Quaternions/3 -> Out Bus Element7/1
  Euler to Quaternions/2 -> Out Bus Element6/1
  Euler to Quaternions/1 -> Out Bus Element5/1
  NED to LLA Transformation/1 -> Out Bus Element9/1
  NED to LLA Transformation/2 -> Out Bus Element10/1
  In Bus Element14/1 -> NED to LLA Transformation/1
  In Bus Element15/1 -> NED to LLA Transformation/2
  In Bus Element16/1 -> NED to LLA Transformation/3
  In Bus Element17/1 -> True Airspeed to Indicated Airspeed/2
  True Airspeed to Indicated Airspeed/1 -> Out Bus Element11/1
  In Bus Element18/1 -> True Airspeed to Indicated Airspeed/1
  In Bus Element19/1 -> Body Axes Rates to Stability Axes Rates/1
  In Bus Element20/1 -> Body Axes Rates to Stability Axes Rates/2
  In Bus Element21/1 -> Body Axes Rates to Stability Axes Rates/3
  Body Axes Rates to Stability Axes Rates/1 -> Out Bus Element12/1
  Body Axes Rates to Stability Axes Rates/2 -> Out Bus Element13/1

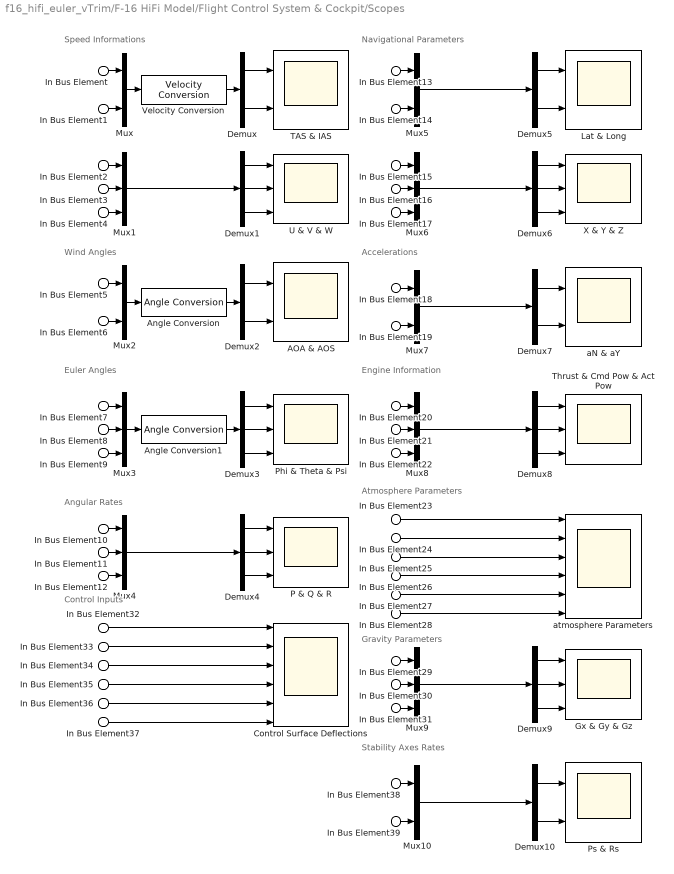
== system f16_hifi_euler_vTrim/F-16 HiFi Model/Flight Control System & Cockpit/Scopes ==
  note: Stability Axes Rates
  note: Speed Informations
  note: Wind Angles
  note: Euler Angles
  note: Angular Rates
  note: Navigational Parameters
  note: Accelerations
  note: Engine Information
  note: Atmosphere Parameters
  note: Gravity Parameters
  note: Control Inputs
  In Bus Element : Inport  PortName=states  Element=tas
  In Bus Element5 : Inport  PortName=states  Element=alpha
  In Bus Element6 : Inport  PortName=states  Element=beta
  In Bus Element7 : Inport  PortName=states  Element=phi
  In Bus Element8 : Inport  PortName=states  Element=theta
  In Bus Element9 : Inport  PortName=states  Element=psi
  In Bus Element10 : Inport  PortName=states  Element=p
  In Bus Element11 : Inport  PortName=states  Element=q
  In Bus Element12 : Inport  PortName=states  Element=r
  In Bus Element15 : Inport  PortName=states  Element=x_e
  In Bus Element16 : Inport  PortName=states  Element=y_e
  In Bus Element17 : Inport  PortName=states  Element=z_e
  In Bus Element22 : Inport  PortName=states  Element=power
  In Bus Element1 : Inport  Port=2  PortName=sensorData  Element=ias
  In Bus Element2 : Inport  Port=2  PortName=sensorData  Element=u
  In Bus Element3 : Inport  Port=2  PortName=sensorData  Element=v
  In Bus Element4 : Inport  Port=2  PortName=sensorData  Element=w
  In Bus Element14 : Inport  Port=2  PortName=sensorData  Element=long
  In Bus Element13 : Inport  Port=2  PortName=sensorData  Element=lat
  In Bus Element18 : Inport  Port=2  PortName=sensorData  Element=aN
  In Bus Element19 : Inport  Port=2  PortName=sensorData  Element=aY
  In Bus Element38 : Inport  Port=2  PortName=sensorData  Element=p_s
  In Bus Element39 : Inport  Port=2  PortName=sensorData  Element=r_s
  In Bus Element20 : Inport  Port=3  PortName=engine  Element=thrust
  In Bus Element21 : Inport  Port=3  PortName=engine  Element=cmdPow
  In Bus Element23 : Inport  Port=4  PortName=atmParam  Element=temp
  In Bus Element24 : Inport  Port=4  PortName=atmParam  Element=rho
  In Bus Element25 : Inport  Port=4  PortName=atmParam  Element=a
  In Bus Element26 : Inport  Port=4  PortName=atmParam  Element=mach
  In Bus Element27 : Inport  Port=4  PortName=atmParam  Element=qbar
  In Bus Element28 : Inport  Port=4  PortName=atmParam  Element=pSta
  In Bus Element29 : Inport  Port=5  PortName=graParam  Element=g_x
  In Bus Element31 : Inport  Port=5  PortName=graParam  Element=g_z
  In Bus Element30 : Inport  Port=5  PortName=graParam  Element=g_y
  In Bus Element32 : Inport  Port=6  PortName=pilotSignals  Element=thrtl
  In Bus Element33 : Inport  Port=6  PortName=pilotSignals  Element=ele
  In Bus Element34 : Inport  Port=6  PortName=pilotSignals  Element=ail
  In Bus Element35 : Inport  Port=6  PortName=pilotSignals  Element=rud
  In Bus Element36 : Inport  Port=6  PortName=pilotSignals  Element=sb
  In Bus Element37 : Inport  Port=6  PortName=pilotSignals  Element=lef
  AOA & AOS : Scope  NumInputPorts=2
  Angle Conversion : aerolibconvert2/Angle Conversion  IU=rad  OU=deg
  Angle Conversion1 : aerolibconvert2/Angle Conversion  IU=rad  OU=deg
  Control Surface Deflections : Scope  NumInputPorts=6
  Demux{,2,5,7,10} (5 alike) : Demux  Outputs=2
  Demux{1,3..4,6,8..9} (6 alike) : Demux  Outputs=3
  Gx & Gy & Gz : Scope  NumInputPorts=3
  Lat & Long : Scope  NumInputPorts=2
  Mux{,2,5,7,10} (5 alike) : Mux  Inputs=2
  Mux{1,3..4,6,8..9} (6 alike) : Mux  Inputs=3
  P & Q & R : Scope  NumInputPorts=3
  Phi & Theta & Psi : Scope  NumInputPorts=3
  Ps & Rs : Scope  NumInputPorts=2
  TAS & IAS : Scope  NumInputPorts=2
  Thrust & Cmd Pow & Act Pow : Scope  NumInputPorts=3
  U & V & W : Scope  NumInputPorts=3
  Velocity Conversion : aerolibconvert2/Velocity Conversion  IU=ft/s  OU=kts
  X & Y & Z : Scope  NumInputPorts=3
  aN & aY : Scope  NumInputPorts=2
  atmosphere Parameters : Scope  NumInputPorts=6
  wires:
  In Bus Element39/1 -> Mux10/2
  Demux10/2 -> Ps & Rs/2
  Mux10/1 -> Demux10/1
  Demux10/1 -> Ps & Rs/1
  In Bus Element38/1 -> Mux10/1
  In Bus Element32/1 -> Control Surface Deflections/1
  In Bus Element33/1 -> Control Surface Deflections/2
  In Bus Element34/1 -> Control Surface Deflections/3
  In Bus Element35/1 -> Control Surface Deflections/4
  In Bus Element36/1 -> Control Surface Deflections/5
  In Bus Element37/1 -> Control Surface Deflections/6
  Demux9/2 -> Gx & Gy & Gz/2
  In Bus Element29/1 -> Mux9/1
  In Bus Element31/1 -> Mux9/3
  Mux9/1 -> Demux9/1
  Demux9/3 -> Gx & Gy & Gz/3
  In Bus Element30/1 -> Mux9/2
  Demux9/1 -> Gx & Gy & Gz/1
  In Bus Element23/1 -> atmosphere Parameters/1
  In Bus Element24/1 -> atmosphere Parameters/2
  In Bus Element25/1 -> atmosphere Parameters/3
  In Bus Element26/1 -> atmosphere Parameters/4
  In Bus Element27/1 -> atmosphere Parameters/5
  In Bus Element28/1 -> atmosphere Parameters/6
  Demux8/2 -> Thrust & Cmd Pow & Act Pow/2
  In Bus Element20/1 -> Mux8/1
  In Bus Element22/1 -> Mux8/3
  Demux8/3 -> Thrust & Cmd Pow & Act Pow/3
  Demux8/1 -> Thrust & Cmd Pow & Act Pow/1
  In Bus Element21/1 -> Mux8/2
  Mux8/1 -> Demux8/1
  In Bus Element18/1 -> Mux7/1
  Mux7/1 -> Demux7/1
  Demux7/2 -> aN & aY/2
  Demux7/1 -> aN & aY/1
  In Bus Element19/1 -> Mux7/2
  Demux6/3 -> X & Y & Z/3
  In Bus Element17/1 -> Mux6/3
  Demux5/2 -> Lat & Long/2
  In Bus Element16/1 -> Mux6/2
  Demux6/2 -> X & Y & Z/2
  Demux6/1 -> X & Y & Z/1
  In Bus Element13/1 -> Mux5/1
  Mux5/1 -> Demux5/1
  In Bus Element14/1 -> Mux5/2
  In Bus Element15/1 -> Mux6/1
  Mux6/1 -> Demux6/1
  Demux5/1 -> Lat & Long/1
  Demux4/2 -> P & Q & R/2
  In Bus Element10/1 -> Mux4/1
  In Bus Element12/1 -> Mux4/3
  Demux4/3 -> P & Q & R/3
  Demux4/1 -> P & Q & R/1
  In Bus Element11/1 -> Mux4/2
  Mux4/1 -> Demux4/1
  Angle Conversion1/1 -> Demux3/1
  In Bus Element8/1 -> Mux3/2
  Demux3/2 -> Phi & Theta & Psi/2
  In Bus Element9/1 -> Mux3/3
  Demux3/3 -> Phi & Theta & Psi/3
  Demux3/1 -> Phi & Theta & Psi/1
  In Bus Element7/1 -> Mux3/1
  Mux3/1 -> Angle Conversion1/1
  Angle Conversion/1 -> Demux2/1
  Demux2/1 -> AOA & AOS/1
  In Bus Element5/1 -> Mux2/1
  Demux2/2 -> AOA & AOS/2
  Mux2/1 -> Angle Conversion/1
  In Bus Element6/1 -> Mux2/2
  Demux1/1 -> U & V & W/1
  Demux1/2 -> U & V & W/2
  Demux1/3 -> U & V & W/3
  Mux1/1 -> Demux1/1
  In Bus Element4/1 -> Mux1/3
  In Bus Element3/1 -> Mux1/2
  In Bus Element2/1 -> Mux1/1
  Demux/1 -> TAS & IAS/1
  Demux/2 -> TAS & IAS/2
  Velocity Conversion/1 -> Demux/1
  Mux/1 -> Velocity Conversion/1
  In Bus Element1/1 -> Mux/2
  In Bus Element/1 -> Mux/1
